simulink model "PID_volts"  (R2018a)
settings: Solver=FixedStepAuto  StartTime=0.0  StopTime=80  RelTol=1e-3
PreLoadFcn:
  | % Plant
  | K0=0.82/0.017;
  | tau0=0.26;
  | N=9;
  | Kpot=1.62;
  | % Sampling period
  | Ts=0.01;
  | 
  | % Desired control specifications
  | Sp=80; % overshoot
  | Fd=0.5; % frequency
  | 
  | % Poles of the second order continuous system that will fulfill the specifications
  | wd=2*pi*Fd ;
  | xi=sqrt((log(Sp/100))^2/(pi^2+log(Sp/100)^2))
  | wn=wd/ sqrt(1-xi^2)
  | s1=-xi*wn+j*wd
  | s2=-xi*wn-j*wd
  | 
  | % Poles of the second order discrete system that will fulfill the specifications
  | p1=exp(Ts* s1 )
  | p2=exp(Ts* s2 )
  | % Fix third pole
  | p3=0.01
  | 
  | % Plant's Z transfere function
  | Ptas=tf([K0*(1/N)],[tau0,1,0]);
  | Ptaz=c2d(Ptas,Ts,'zoh');
  | 
  | % Denominator and numerator coefficients
  | [Nz ,Dz]= tfdata(Ptaz,'v')
  | a1=Nz(2);
  | a0=Nz(3);
  | b1=Dz(2);
  | b0=Dz(3);
  | 
  | % A and B matrix definitions
  | A=[-1 -a1 -a1 -a1 ; p2+p3+p1 a1-a0 -a1-a0 -a0+2*a1 ; ...
  |    -p1*p2-p3*p1-p2*p3 a0 -a0 2*a0-a1 ; p1*p2*p3 0 0 -a0 ] ;
  | b=[p1+p2+p3-1+b1 ; -p1*p2-p3*p1-p3*p2+b0-b1 ; p1*p2*p3-b0 ; 0 ] ;
  | 
  | % x vector's determination of the controller
  | x=inv(A)*b ;
  | 
  | p4=x(1)
  | Kp=x(2)
  | Ki=(2/Ts)*x(3)
  | Kd=Ts*x(4)
  | pawd=0.2;
  | Kaw=1/Ki;
  | 
  | % Poles dominance calculation
  | dominancia=log(abs(p4))/log(abs(p1))
undefined symbols (not defined in the file or in its folder): DiscIntNeverNeededParam
libraries: arduinolib x4, simulink x2
settings Model: SimulationMode=external  ExtModeTrigDuration=2  Creator=Eneko Lerma  LastModifiedBy=Eneko Lerma
settings OptimizationCC: EnhancedBackFolding=on  PassReuseOutputArgsAs=Individual arguments  MaxStackSize=64  OptimizeBlockOrder=speed  DifferentSizesBufferReuse=on  OptimizationCustomize=off
settings DebuggingCC: ParameterPrecisionLossMsg=none  ParameterTunabilityLossMsg=error
settings HardwareCC: ProdBitPerPointer=32  ProdBitPerSizeT=32  ProdBitPerPtrDiffT=32  ProdLargestAtomicInteger=Long  ProdLargestAtomicFloat=Double  ProdWordSize=32  ProdHWDeviceType=ARM Compatible->ARM Cortex
settings SFSimCC: MATLABDynamicMemAlloc=off
settings RTWCC: SystemTargetFile=ert.tlc  HardwareBoard=Arduino Due  TLCOptions=-aInlineSetEventsForThisBaseRateFcn=TLC_FALSE -aSuppressMultiTaskScheduler=TLC_FALSE -aRateBasedStepFcn=1  TemplateMakefile=ert_default_tmf  GenerateReport=on  Toolchain=Arduino ARM  BuildConfiguration=Faster Runs  IncludeHyperlinkInReport=on  LaunchReport=on  GenerateTraceInfo=on  GenerateTraceReport=on  GenerateTraceReportSl=on  GenerateTraceReportSf=on  GenerateTraceReportEml=on
settings RTWCC: CustomTerminator=|
  | writeDigitalPin((uint8_T)3, 0);
  | writeDigitalPin((uint8_T)5, 0);
settings CodeAppCC: ForceParamTrailComments=on  IgnoreCustomStorageClasses=off  OperatorAnnotations=on  SimulinkDataObjDesc=on  SFDataObjDesc=on  InsertBlockDesc=on
settings ERTTargetCC: SupportContinuousTime=on  SupportVariableSizeSignals=on

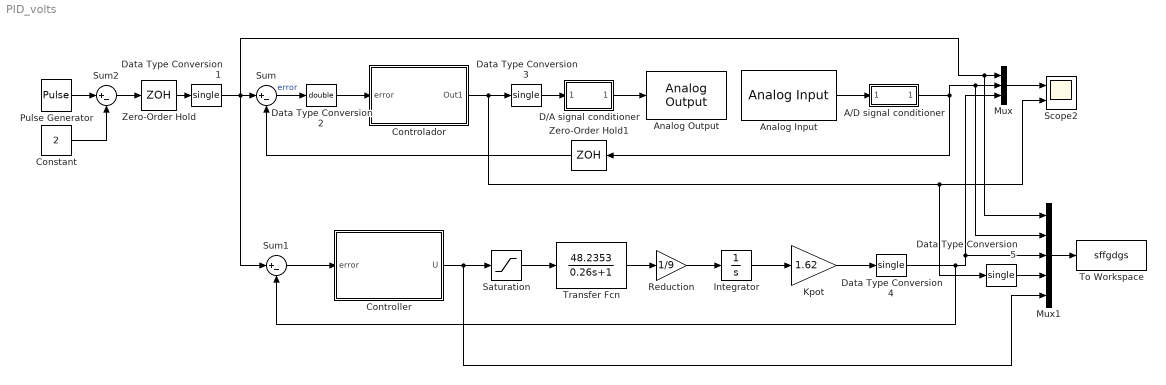
== system PID_volts ==
  A/D signal conditioner : Subsystem
  Analog Input : arduinolib/Analog Input  pinNumber=1  ReadResultsOnly=off  ConversionTriggerSource=Software  ExternalTriggerType=uint32(0)  OutputDataType=uint16  EnableConversionCompleteNotify=off  EnableOuputStatus=off  SampleTime=0.005  blockPlatform=arduino
  Analog Output : arduinolib/Analog Output  DACpin=DAC1  blockPlatform=arduino
      settings: SourceProductName=Simulink Support Package for Arduino Hardware  SourceProductBaseCode=ARDUINO
  Constant : Constant  Value=2
  Controlador : Subsystem
  Controller : Subsystem
  D/A signal conditioner : Subsystem
  Data Type Conversion{1,3..5} (4 alike) : DataTypeConversion  OutDataTypeStr=single
  Data Type Conversion2 : DataTypeConversion  OutDataTypeStr=double
  Integrator : Integrator
  Kpot : Gain  Gain=1.62  OutDataTypeStr=single
  Mux : Mux  Inputs=3
  Mux1 : Mux  Inputs=5
  Pulse Generator : DiscretePulseGenerator  PulseType=Time based  Amplitude=4  Period=20  PulseWidth=50
  Reduction : Gain  Gain=1/9  OutDataTypeStr=double
  Saturation : Saturate  UpperLimit=5  LowerLimit=-5  OutDataTypeStr=double
  Scope2 : Scope  NumInputPorts=2
  Sum : Sum  Inputs=|+-  AccumDataTypeStr=single
  Sum1 : Sum  Inputs=|+-  AccumDataTypeStr=single
  Sum2 : Sum  Inputs=|+-
  To Workspace : ToWorkspace  VariableName=sffgdgs  SaveFormat=Structure With Time  SampleTime=-1
  Transfer Fcn : TransferFcn  Numerator=[48.2353]  Denominator=[0.26 1]
  Zero-Order Hold : ZeroOrderHold  SampleTime=Ts
  Zero-Order Hold1 : ZeroOrderHold  SampleTime=Ts
  wires:
  Mux/1 -> Scope2/1
  A/D signal conditioner/1(" ") -> Zero-Order Hold1/1, Mux1/2, Mux/2
  Sum/1 -> Data Type Conversion2/1  "error"
  D/A signal conditioner/1(" ") -> Analog Output/1
  Zero-Order Hold/1 -> Data Type Conversion1/1
  Zero-Order Hold1/1 -> Sum/2
  Data Type Conversion3/1 -> D/A signal conditioner/1("  ")
  Analog Input/1 -> A/D signal conditioner/1("  ")
  Data Type Conversion1/1 -> Sum1/1, Mux1/1, Mux/1, Sum/1
  Sum2/1 -> Zero-Order Hold/1
  Controlador/1(Out1) -> Data Type Conversion5/1, Scope2/2, Data Type Conversion3/1
  Data Type Conversion2/1 -> Controlador/1(error)
  Sum1/1 -> Controller/1(error)
  Integrator/1 -> Kpot/1
  Transfer Fcn/1 -> Reduction/1
  Saturation/1 -> Transfer Fcn/1
  Reduction/1 -> Integrator/1
  Kpot/1 -> Data Type Conversion4/1
  Data Type Conversion4/1 -> Sum1/2, Mux1/3, Mux/3
  Pulse Generator/1 -> Sum2/1
  Constant/1 -> Sum2/2
  Mux1/1 -> To Workspace/1
  Data Type Conversion5/1 -> Mux1/4
  Controller/1(U) -> Mux1/5, Saturation/1

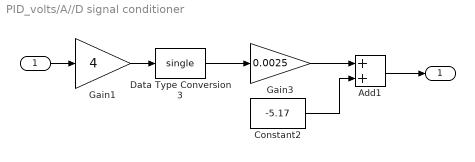
== system PID_volts/A//D signal conditioner ==
  "  " : Inport  OutDataTypeStr=uint16
  Add1 : Sum  AccumDataTypeStr=single
  Constant2 : Constant  Value=-5.17  OutDataTypeStr=single
  Data Type Conversion3 : DataTypeConversion  OutDataTypeStr=single
  Gain1 : Gain  Gain=4  OutDataTypeStr=uint16
  Gain3 : Gain  Gain=0.0025  OutDataTypeStr=single
  " " : Outport  OutDataTypeStr=single
  wires:
  Add1/1 -> " "/1
  Constant2/1 -> Add1/2
  Gain3/1 -> Add1/1
  Data Type Conversion3/1 -> Gain3/1
  "  "/1 -> Gain1/1
  Gain1/1 -> Data Type Conversion3/1

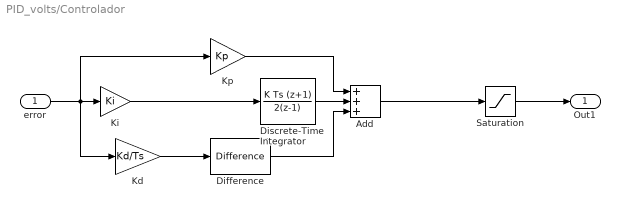
== system PID_volts/Controlador ==
  error : Inport
  Add : Sum  Inputs=+++  AccumDataTypeStr=single
  Difference : simulink/Discrete/Difference  ICPrevInput=0.0  OutMin=[]  OutMax=[]  OutDataType=fixdt(1, 16)  OutScaling=2^-10  DoSatur=off
  Discrete-Time Integrator : DiscreteIntegrator  IntegratorMethod=Integration: Trapezoidal  SampleTime=Ts  ICPrevOutput=DiscIntNeverNeededParam  ICPrevScaledInput=DiscIntNeverNeededParam
  Kd : Gain  Gain=Kd/Ts
  Ki : Gain  Gain=Ki
  Kp : Gain  Gain=Kp
  Saturation : Saturate  UpperLimit=5  LowerLimit=-5  OutDataTypeStr=double
  Out1 : Outport  OutDataTypeStr=double
  wires:
  Difference/1 -> Add/3
  Kp/1 -> Add/1
  Discrete-Time Integrator/1 -> Add/2
  Kd/1 -> Difference/1
  Ki/1 -> Discrete-Time Integrator/1
  Add/1 -> Saturation/1
  Saturation/1 -> Out1/1
  error/1 -> Ki/1, Kp/1, Kd/1

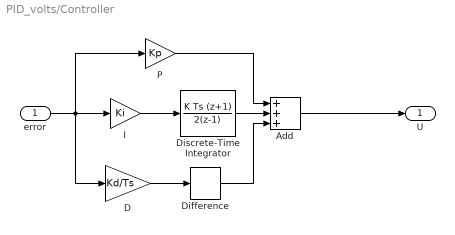
== system PID_volts/Controller ==
  error : Inport
  Add : Sum  Inputs=+++  AccumDataTypeStr=single
  D : Gain  Gain=Kd/Ts
  Difference : simulink/Discrete/Difference  ICPrevInput=0.0  OutMin=[]  OutMax=[]  OutDataType=fixdt(1, 16)  OutScaling=2^-10  DoSatur=off
  Discrete-Time Integrator : DiscreteIntegrator  IntegratorMethod=Integration: Trapezoidal  SampleTime=Ts  ICPrevOutput=DiscIntNeverNeededParam  ICPrevScaledInput=DiscIntNeverNeededParam
  I : Gain  Gain=Ki
  P : Gain  Gain=Kp
  U : Outport
  wires:
  Difference/1 -> Add/3
  Discrete-Time Integrator/1 -> Add/2
  error/1 -> P/1, I/1, D/1
  I/1 -> Discrete-Time Integrator/1
  P/1 -> Add/1
  D/1 -> Difference/1
  Add/1 -> U/1

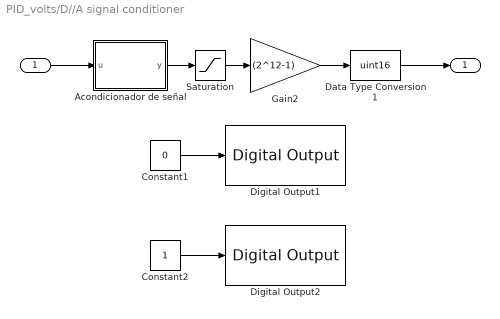
== system PID_volts/D//A signal conditioner ==
  "  " : Inport  OutDataTypeStr=single
  Acondicionador de señal : MATLAB Function  TreatAsAtomicUnit=on
  Constant1 : Constant  Value=0
  Constant2 : Constant
  Data Type Conversion1 : DataTypeConversion  OutDataTypeStr=uint16
  Digital Output1 : arduinolib/Digital Output  pinNumber=5  blockPlatform=arduino
  Digital Output2 : arduinolib/Digital Output  pinNumber=3  blockPlatform=arduino
  Gain2 : Gain  Gain=(2^12-1)  OutDataTypeStr=single
  Saturation : Saturate  UpperLimit=1  LowerLimit=0  OutDataTypeStr=single
  " " : Outport  OutDataTypeStr=uint16
  wires:
  Gain2/1 -> Data Type Conversion1/1
  "  "/1 -> Acondicionador de señal/1(u)
  Acondicionador de señal/1(y) -> Saturation/1
  Data Type Conversion1/1 -> " "/1
  Saturation/1 -> Gain2/1
  Constant1/1 -> Digital Output1/1
  Constant2/1 -> Digital Output2/1

== matlab function PID_volts/D//A signal conditioner/Acondicionador de señal ==
  data: u input; y output
function y = fcn(u)
y =0.0961*u+0.5099;
